simulink model "esquema"  (R2014b)
settings: Solver=ode5  StartTime=0.0  StopTime=Te  FixedStep=Tm  RelTol=1e-3
StopFcn:
  | %salida(simout)
values from neighbouring files (symbols this model uses):
  Dp = 0    [globales.mat]
  Dv = 0    [globales.mat]
  Ip = 0    [globales.mat]
  Iv = 0    [globales.mat]
  Ka = 0    [globales.mat]
  Kbp = 0    [globales.mat]
  Kbv = 0    [globales.mat]
  Kv = 0    [globales.mat]
  Np = 1    [globales.mat]
  Nv = 1    [globales.mat]
  Pp = 0.1    [globales.mat]
  Pv = 0.1    [globales.mat]
  Tm = 0.5    [globales.mat]
undefined symbols (not defined in the file or in its folder): A, B
undefined symbols (not defined in the file): Fcdp, Fcdv, Fcp, Fcv
settings Model: ExtModeTrigDuration=100000  Creator=Equipo-Servo  LastModifiedBy=E. Rubio
settings DebuggingCC: UnderspecifiedInitializationDetection=Classic  MergeDetectMultiDrivingBlocksExec=none  StateNameClashWarn=warning
settings HardwareCC: ProdIntDivRoundTo=Zero  ProdEndianess=LittleEndian  ProdHWDeviceType=Generic->32-bit x86 compatible
settings RTWCC: SystemTargetFile=rtwin.tlc  TemplateMakefile=rtwin.tmf  Description=Real-Time Windows Target  ProcessScript=rtwin_make_rtw_hook  RTWCompilerOptimization=On
settings CodeAppCC: MaxIdLength=95
settings RTWinTargetCC: TargetLibSuffix=_rtwin.lib  TargetPreCompLibLocation=C:\Program Files\MATLAB\R2014b\toolbox\rtw\targets\rtwin\lib\win64

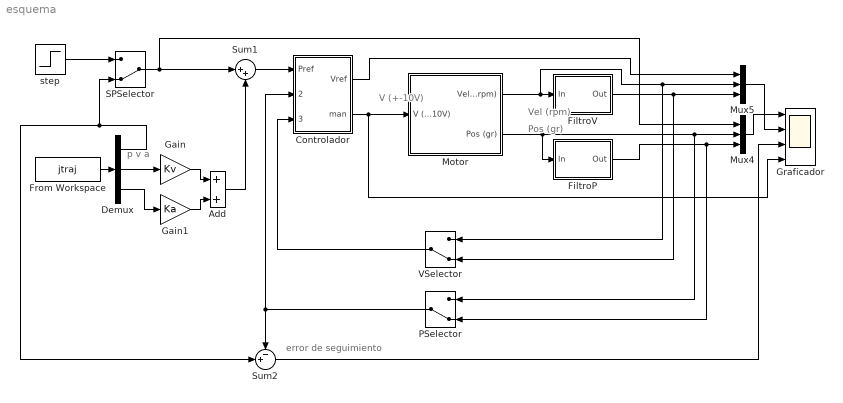
== system esquema ==
  note: p
      |
      | v
      |
      | a
  note: error de seguimiento
  note: Vel
      | (rpm)
  note: Pos
      | (gr)
  note: V (+-10V)
  Add : Sum
  Controlador : Subsystem  mask{T=Tm, Pp=Pp, Ip=Ip, Kbp=Kbp, Dp=Dp, Fcdp=Fcdp, Pv=Pv, Iv=Iv, Kbv=Kbv, Dv=Dv, Fcdv=Fcdv}
      mask prompts: T "Período de muestreo"; Kbp "Kbp (anti windup)"; Fcdp "Fcdp (Hz)"; Kbv "Kbv (anti windup)"; Fcdv "Fcdv (Hz)"
      mask init:
      | Np = 2*pi*Fcdp;
      | Nv = 2*pi*Fcdv;
  Demux : Demux  Outputs=3
  FiltroP : Subsystem  mask{N=Np, Fc=Fcp, Fm=1/Tm}
      mask prompts: N "Orden del filtro (Butterworth)"; Fc "Frecuencia de corte (Fc<Fm/2)"; Fm "Frecuencia de muestreo"
      mask init:
      | Fn = Fm/2;   % Frecuencia de Nyquist
      | [B,A] = butter(N,Fc/Fn);
  FiltroV : Subsystem  mask{N=Nv, Fc=Fcv, Fm=1/Tm}
      mask prompts: N "Orden del filtro (Butterworth)"; Fc "Frecuencia de corte (Fc<Fm/2)"; Fm "Frecuencia de muestreo"
      mask init:
      | Fn = Fm/2;   % Frecuencia de Nyquist
      | [B,A] = butter(N,Fc/Fn);
  From Workspace : FromWorkspace  VariableName=jtraj  SampleTime=0
  Gain : Gain  Gain=Kv
  Gain1 : Gain  Gain=Ka
  Graficador : Scope  NumInputPorts=4
      settings: TimeRange=10  YMin=-100~-100~-30~-10  YMax=100~100~30~10  SampleTime=Tm
  Motor : Subsystem
  Mux4 : Mux  Inputs=3
  Mux5 : Mux  Inputs=3
  PSelector : ManualSwitch  CurrentSetting=0
  SPSelector : ManualSwitch  CurrentSetting=0
  Sum1 : Sum  Inputs=|++
  Sum2 : Sum  Inputs=-+|
  VSelector : ManualSwitch  CurrentSetting=0
  step : Step  Time=5  Before=-50  After=50  SampleTime=0.01
  wires:
  Motor/2(Pos (gr)) -> FiltroP/1(In), Mux4/2, PSelector/1
  SPSelector/1 -> Sum1/1, Mux4/1
  FiltroP/1(Out) -> Mux4/3, PSelector/2
  PSelector/1 -> Controlador/2(Pmed), Sum2/1
  Controlador/2(man) -> Motor/1(V (+-10V)), Graficador/4
  Motor/1(Vel (rpm)) -> VSelector/1, Mux5/2, FiltroV/1(In)
  FiltroV/1(Out) -> VSelector/2, Mux5/3
  Controlador/1(Vref) -> Mux5/1
  VSelector/1 -> Controlador/3(Vmed)
  Mux4/1 -> Graficador/1
  Mux5/1 -> Graficador/2
  step/1 -> SPSelector/1
  From Workspace/1 -> Demux/1
  Demux/2 -> Gain/1
  Demux/3 -> Gain1/1
  Gain/1 -> Add/1
  Gain1/1 -> Add/2
  Demux/1 -> Sum2/2, SPSelector/2
  Add/1 -> Sum1/2
  Sum1/1 -> Controlador/1(Pref)
  Sum2/1 -> Graficador/3

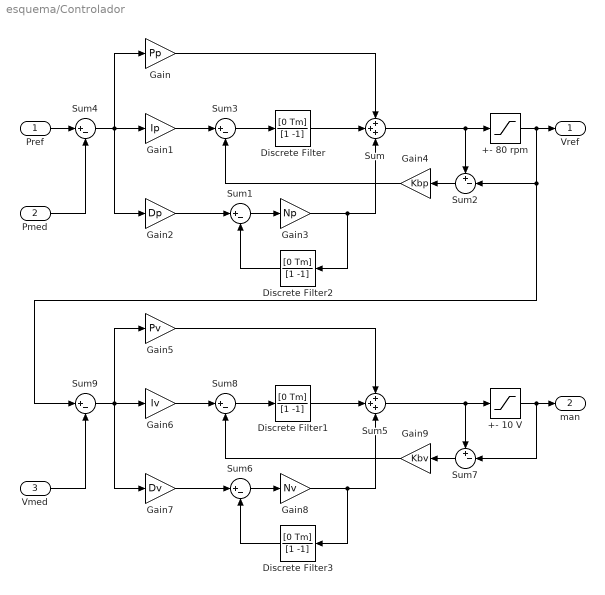
== system esquema/Controlador ==
  Pref : Inport
  Pmed : Inport  Port=2
  Vmed : Inport  Port=3
  +- 10 V : Saturate  UpperLimit=10  LowerLimit=-10
  +- 80 rpm : Saturate  UpperLimit=80  LowerLimit=-80
  Discrete Filter{,1..3} (4 alike) : DiscreteFilter  Numerator=[0 Tm]  Denominator=[1 -1]
  Gain : Gain  Gain=Pp
  Gain1 : Gain  Gain=Ip
  Gain2 : Gain  Gain=Dp
  Gain3 : Gain  Gain=Np
  Gain4 : Gain  Gain=Kbp
  Gain5 : Gain  Gain=Pv
  Gain6 : Gain  Gain=Iv
  Gain7 : Gain  Gain=Dv
  Gain8 : Gain  Gain=Nv
  Gain9 : Gain  Gain=Kbv
  Sum : Sum  Inputs=+++
  Sum{1,3..4,6,8..9} (6 alike) : Sum  Inputs=|+-
  Sum2 : Sum  Inputs=+-|
  Sum5 : Sum  Inputs=+++
  Sum7 : Sum  Inputs=+-|
  Vref : Outport
  man : Outport  Port=2
  wires:
  Sum/1 -> Sum2/1, +- 80 rpm/1
  Gain/1 -> Sum/1
  Discrete Filter/1 -> Sum/2
  Pref/1 -> Sum4/1
  Sum1/1 -> Gain3/1
  Gain2/1 -> Sum1/1
  Discrete Filter2/1 -> Sum1/2
  Gain3/1 -> Discrete Filter2/1, Sum/3
  Sum2/1 -> Gain4/1
  Sum3/1 -> Discrete Filter/1
  Gain1/1 -> Sum3/1
  Gain4/1 -> Sum3/2
  Sum4/1 -> Gain2/1, Gain/1, Gain1/1
  Pmed/1 -> Sum4/2
  Sum5/1 -> +- 10 V/1, Sum7/1
  +- 10 V/1 -> man/1, Sum7/2
  Gain5/1 -> Sum5/1
  Discrete Filter1/1 -> Sum5/2
  +- 80 rpm/1 -> Sum9/1, Sum2/2, Vref/1
  Sum6/1 -> Gain8/1
  Gain7/1 -> Sum6/1
  Discrete Filter3/1 -> Sum6/2
  Gain8/1 -> Discrete Filter3/1, Sum5/3
  Sum7/1 -> Gain9/1
  Sum8/1 -> Discrete Filter1/1
  Gain6/1 -> Sum8/1
  Gain9/1 -> Sum8/2
  Sum9/1 -> Gain7/1, Gain6/1, Gain5/1
  Vmed/1 -> Sum9/2

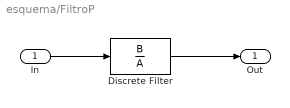
== system esquema/FiltroP ==
  In : Inport
  Discrete Filter : DiscreteFilter  Numerator=B  Denominator=A  SampleTime=1/Fm
  Out : Outport
  wires:
  Discrete Filter/1 -> Out/1
  In/1 -> Discrete Filter/1

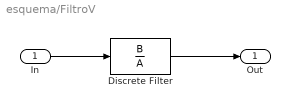
== system esquema/FiltroV ==
  In : Inport
  Discrete Filter : DiscreteFilter  Numerator=B  Denominator=A  SampleTime=1/Fm
  Out : Outport
  wires:
  In/1 -> Discrete Filter/1
  Discrete Filter/1 -> Out/1

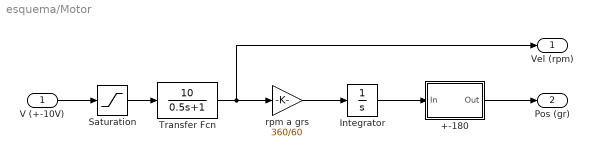
== system esquema/Motor ==
  V (+-10V) : Inport
  +-180 : Subsystem
  Integrator : Integrator  InitialCondition=180  UpperSaturationLimit=180  LowerSaturationLimit=-180
  Saturation : Saturate  UpperLimit=10  LowerLimit=-10
  Transfer Fcn : TransferFcn  Numerator=[10]  Denominator=[0.5 1]
  rpm a grs : Gain  Gain=360/60
  Vel (rpm) : Outport
  Pos (gr) : Outport  Port=2
  wires:
  V (+-10V)/1 -> Saturation/1
  Transfer Fcn/1 -> Vel (rpm)/1, rpm a grs/1
  Integrator/1 -> +-180/1(In)
  Saturation/1 -> Transfer Fcn/1
  +-180/1(Out) -> Pos (gr)/1
  rpm a grs/1 -> Integrator/1

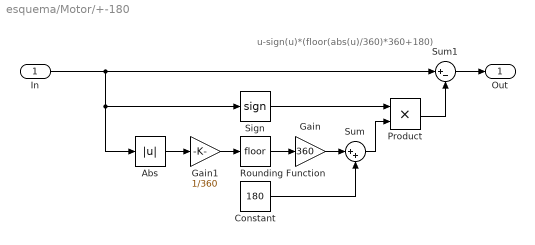
== system esquema/Motor/+-180 ==
  note: u-sign(u)*(floor(abs(u)/360)*360+180)
  In : Inport
  Abs : Abs
  Constant : Constant  Value=180
  Gain : Gain  Gain=360
  Gain1 : Gain  Gain=1/360
  Product : Product
  Rounding Function : Rounding
  Sign : Signum
  Sum : Sum  Inputs=|++
  Sum1 : Sum  Inputs=|+-
  Out : Outport
  wires:
  Sum/1 -> Product/2
  Constant/1 -> Sum/2
  Sign/1 -> Product/1
  Gain1/1 -> Rounding Function/1
  Gain/1 -> Sum/1
  Rounding Function/1 -> Gain/1
  Sum1/1 -> Out/1
  Abs/1 -> Gain1/1
  Product/1 -> Sum1/2
  In/1 -> Abs/1, Sign/1, Sum1/1
